simulink model "pedal_post_logic_and_sensor_wrapper"  (R2024b)
settings: Solver=FixedStepDiscrete  StartTime=0.0  StopTime=1  RelTol=1e-3
Description:
  | Temporary wrapper for PIL simulation
settings Model: Creator=Ahmed  LastModifiedBy=Ahmed
settings OptimizationCC: DefaultParameterBehavior=Inlined  UseDivisionForNetSlopeComputation=on  GainParamInheritBuiltInType=on  UseFloatMulNetSlope=on  InlineInvariantSignals=on  PassReuseOutputArgsAs=Individual arguments  ZeroExternalMemoryAtStartup=off  ZeroInternalMemoryAtStartup=off  NoFixptDivByZeroProtection=on  EfficientFloat2IntCast=on  LifeSpan=1  OptimizeBlockOrder=speed  DifferentSizesBufferReuse=on  EfficientTunableParamExpr=on
settings DebuggingCC: ParameterTunabilityLossMsg=error
settings HardwareCC: ProdBitPerInt=16  ProdBitPerPointer=16  ProdBitPerSizeT=16  ProdBitPerPtrDiffT=16  ProdLargestAtomicFloat=None  ProdWordSize=8  ProdLongLongMode=on  ProdHWDeviceType=Atmel->AVR
settings SFSimCC: MATLABDynamicMemAlloc=off
settings RTWCC: Description=Embedded Coder  SystemTargetFile=ert.tlc  TemplateMakefile=ert_default_tmf  PortableWordSizes=on
settings CodeAppCC: ForceParamTrailComments=on  IgnoreCustomStorageClasses=off  OperatorAnnotations=on  SimulinkDataObjDesc=on  SFDataObjDesc=on  CustomSymbolStrGlobalVar=rt$N$M  CustomSymbolStrType=$N$M  CustomSymbolStrFcn=$N$M$F  CustomSymbolStrMacro=$N$M  InsertBlockDesc=on
settings ERTTargetCC: TargetLangStandard=C99 (ISO)  GenerateSampleERTMain=on  IncludeMdlTerminateFcn=off  CombineSignalStateStructs=on  SupportComplex=off  SupportContinuousTime=on  ERTCustomFileTemplate=example_file_process.tlc  ERTFilePackagingFormat=CompactWithDataFile

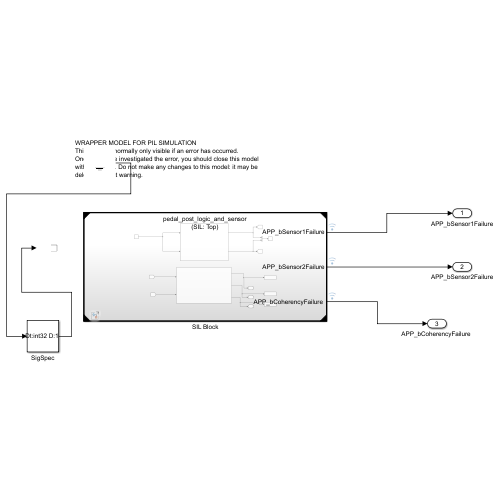
[thumbnail: Simulink's stored preview of the top-level diagram]
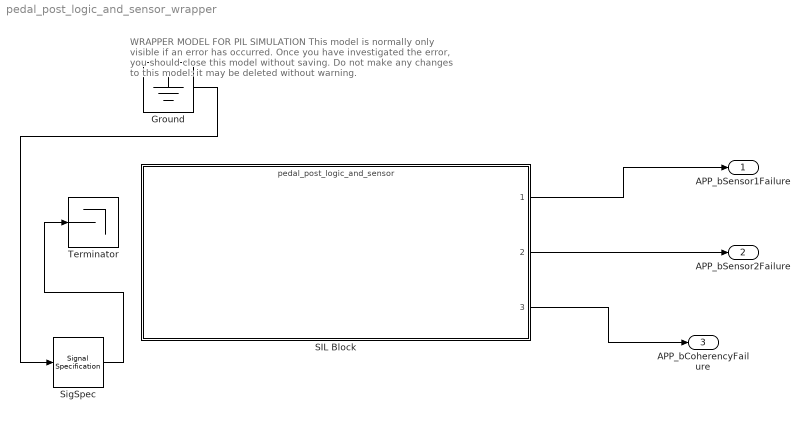
== system pedal_post_logic_and_sensor_wrapper ==
  note: WRAPPER MODEL FOR PIL SIMULATION
      | This model is normally only visible if an error has occurred.
      | Once you have investigated the error, you should close this model
      | without saving. Do not make any changes to this model: it may be
      | deleted without warning.
  Ground : Ground
  SIL Block : ModelReference  ModelNameDialog=pedal_post_logic_and_sensor  SimulationMode=Software-in-the-loop (SIL)  CodeInterface=Top model  ModelReferenceVersion=1.9
  SigSpec : SignalSpecification  OutDataTypeStr=int32  Dimensions=1
  Terminator : Terminator
  APP_bSensor1Failure : Outport
  APP_bSensor2Failure : Outport  Port=2
  "APP_bCoherencyFailure " : Outport  Port=3
  wires:
  SIL Block/1 -> APP_bSensor1Failure/1
  SIL Block/2 -> APP_bSensor2Failure/1
  SIL Block/3 -> "APP_bCoherencyFailure "/1
  Ground/1 -> SigSpec/1
  SigSpec/1 -> Terminator/1
